simulink model "cascadedadrnmpcnofuzzyobs"  (R2024b)
settings: Solver=FixedStepDiscrete  StartTime=0.0  StopTime=80000  FixedStep=0.05  RelTol=1e-3  EnableMultiTasking=on
StartFcn:
  | tic
StopFcn:
  | ttt2=toc
undefined symbols (not defined in the file or in its folder): Force, Torque
libraries: robotlib x12
settings Model: SimulationMode=accelerator  PacingRate=0.010000  Creator=xiejingdong  LastModifiedBy=lenovo
settings SolverCC: ConcurrentTasks=on  AlgebraicLoopSolver=TrustRegion
settings DataIOCC: ReturnWorkspaceOutputs=off
settings DebuggingCC: UnconnectedInputMsg=warning  UnconnectedOutputMsg=warning  UnconnectedLineMsg=warning
settings ModelReferenceCC: EnableRefExpFcnMdlSchedulingChecks=on
settings RTWCC: GPUComputeCapability=3.5  DLArmComputeVersion=19.05

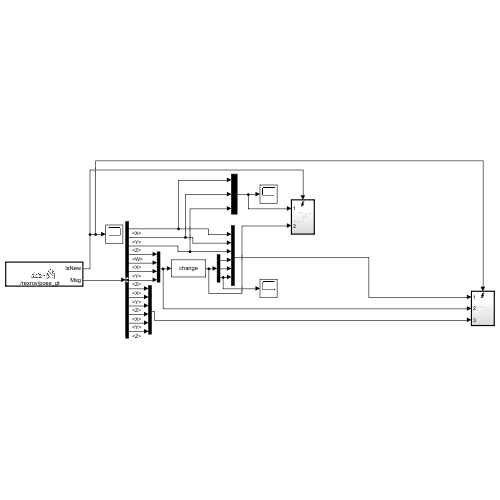
[thumbnail: Simulink's stored preview of the top-level diagram]
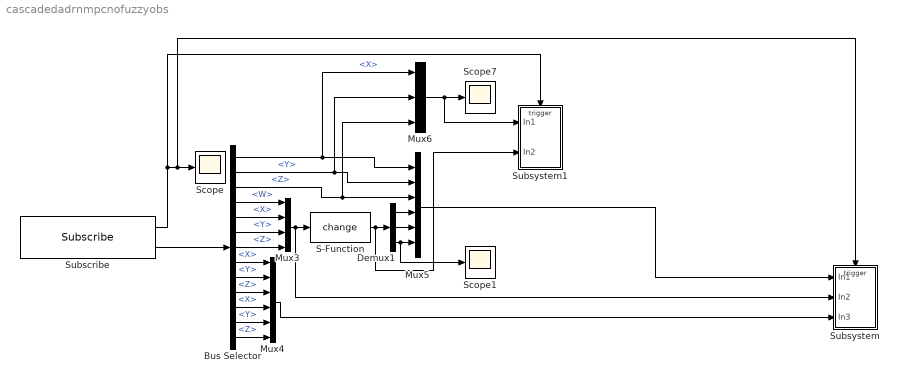
== system cascadedadrnmpcnofuzzyobs ==
  Bus Selector : BusSelector  OutputSignals=Pose.Pose.Position.X,Pose.Pose.Position.Y,Pose.Pose.Position.Z,Pose.Pose.Orientation.W,Pose.Pose.Orientation.X,Pose.Pose.Orientation.Y,Pose.Pose.Orientation.Z,Twist.Twist.Linear.X,Twist.Twist.Linear.Y,Twist.Twist.Linear.Z,Twist.Twist.Angular.X,Twist.Twist.Angular.Y,Twist.Twist.Angular.Z
  Demux1 : Demux  Outputs=3
  Mux3 : Mux
  Mux4 : Mux  Inputs=6
  Mux5 : Mux  Inputs=6
  Mux6 : Mux  Inputs=3
  S-Function : S-Function  FunctionName=change  SFunctionDeploymentMode=off  EnableBusSupport=off
  Scope : Scope
  Scope1 : Scope
  Scope7 : Scope
  Subscribe : robotlib/Subscribe  topicSource=Select from ROS network  topic=/rexrov/pose_gt  messageType=nav_msgs/Odometry  SampleTime=-1  legacyBusStruct=off  messageQueueLength=1
  Subsystem : Subsystem
  Subsystem1 : Subsystem
  wires:
  Subscribe/1 -> Subsystem1/Trigger, Subsystem/Trigger, Scope/1
  Subscribe/2 -> Bus Selector/1
  Bus Selector/4 -> Mux3/1  "<W>"
  Bus Selector/5 -> Mux3/2  "<X>"
  Bus Selector/6 -> Mux3/3  "<Y>"
  Bus Selector/7 -> Mux3/4  "<Z>"
  Bus Selector/8 -> Mux4/1  "<X>"
  Bus Selector/11 -> Mux4/4  "<X>"
  Bus Selector/10 -> Mux4/3  "<Z>"
  Bus Selector/9 -> Mux4/2  "<Y>"
  Bus Selector/12 -> Mux4/5  "<Y>"
  Bus Selector/13 -> Mux4/6  "<Z>"
  Mux3/1 -> Subsystem/2(In2), S-Function/1
  S-Function/1 -> Subsystem1/2(In2), Demux1/1
  Demux1/3 -> Scope1/1, Mux5/6
  Demux1/2 -> Mux5/5
  Demux1/1 -> Mux5/4
  Bus Selector/3 -> Mux6/3, Mux5/3  "<Z>"
  Bus Selector/2 -> Mux6/2, Mux5/2  "<Y>"
  Bus Selector/1 -> Mux6/1, Mux5/1  "<X>"
  Mux6/1 -> Subsystem1/1(In1), Scope7/1
  Mux5/1 -> Subsystem/1(In1)
  Mux4/1 -> Subsystem/3(In3)

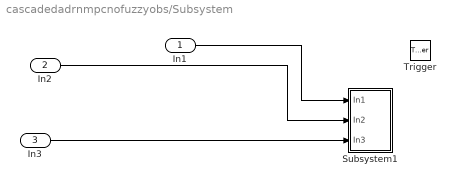
== system cascadedadrnmpcnofuzzyobs/Subsystem ==
  In1 : Inport
  In2 : Inport  Port=2
  In3 : Inport  Port=3
  Trigger : TriggerPort  VariantControl=(inherit)  PortDimensions=1
  Subsystem1 : Subsystem
  wires:
  In1/1 -> Subsystem1/1(In1)
  In2/1 -> Subsystem1/2(In2)
  In3/1 -> Subsystem1/3(In3)

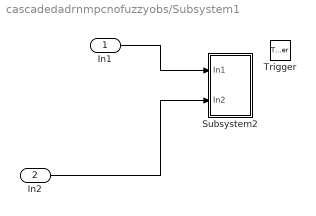
== system cascadedadrnmpcnofuzzyobs/Subsystem1 ==
  In1 : Inport
  In2 : Inport  Port=2
  Trigger : TriggerPort  VariantControl=(inherit)  PortDimensions=1
  Subsystem2 : Subsystem
  wires:
  In2/1 -> Subsystem2/2(In2)
  In1/1 -> Subsystem2/1(In1)

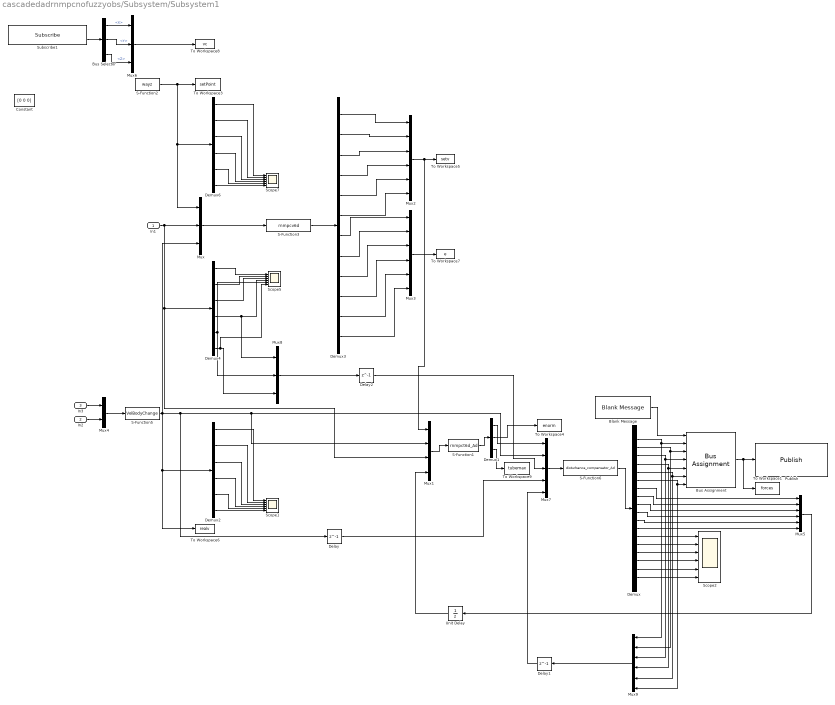
== system cascadedadrnmpcnofuzzyobs/Subsystem/Subsystem1 ==
  In1 : Inport
  In2 : Inport  Port=2
  In3 : Inport  Port=3
  Blank Message : robotlib/Blank Message  messageClass=Message  entityType=geometry_msgs/Wrench  messageType=geometry_msgs/Wrench  SampleTime=-1  legacyBusStruct=off
  Bus Assignment : BusAssignment  AssignedSignals=Force.X,Force.Y,Force.Z,Torque.X,Torque.Y,Torque.Z
  Bus Selector : BusSelector  OutputSignals=Twist.Linear.X,Twist.Linear.Y,Twist.Linear.Z
  Constant : Constant  Value=[0 0 0]
  Delay : Delay  DelayLength=1  InitialCondition=0
  Delay1 : Delay  DelayLength=1  InitialCondition=0
  Delay2 : Delay  DelayLength=1  InitialCondition=0
  Demux : Demux  Outputs=18
  Demux1 : Demux  Outputs=3
  Demux2 : Demux  Outputs=6
  Demux3 : Demux  Outputs=12
  Demux4 : Demux  Outputs=6
  Demux6 : Demux  Outputs=6
  Mux : Mux  Inputs=3
  Mux1 : Mux
  Mux{2..3,5,9} (4 alike) : Mux  Inputs=6
  Mux4 : Mux  Inputs=2
  Mux6 : Mux  Inputs=3
  Mux7 : Mux  Inputs=5
  Mux8 : Mux  Inputs=3
  Publish : robotlib/Publish  topicSource=Select from ROS network  topic=/rexrov/thruster_manager/input  messageType=geometry_msgs/Wrench  legacyBusStruct=off  messageQueueLength=1
  S-Function1 : S-Function  FunctionName=rnmpct6d_Ad  Parameters=0  SFunctionDeploymentMode=off  EnableBusSupport=off
  S-Function2 : S-Function  FunctionName=wayz  SFunctionDeploymentMode=off  EnableBusSupport=off
  S-Function3 : S-Function  FunctionName=rnmpcv6d  Parameters=0  SFunctionDeploymentMode=off  EnableBusSupport=off
  S-Function5 : S-Function  FunctionName=VelBodyChange  SFunctionDeploymentMode=off  EnableBusSupport=off
  S-Function6 : S-Function  FunctionName=disturbance_compensator_Ad  SFunctionDeploymentMode=off  EnableBusSupport=off
  Scope{1..2,5,7} (4 alike) : Scope  NumInputPorts=6
  Subscribe1 : robotlib/Subscribe  topicSource=Select from ROS network  topic=/hydrodynamics/current_velocity  messageType=geometry_msgs/TwistStamped  SampleTime=-1  legacyBusStruct=off  messageQueueLength=1
  To Workspace1 : ToWorkspace  VariableName=forces  SaveFormat=Timeseries  SampleTime=-1
  To Workspace3 : ToWorkspace  VariableName=setPoint  SampleTime=-1
      settings: Save2DSignal=2-D array (concatenate along first dimension)
  To Workspace4 : ToWorkspace  VariableName=enorm  SampleTime=-1
      settings: Save2DSignal=2-D array (concatenate along first dimension)
  To Workspace5 : ToWorkspace  VariableName=setv  SampleTime=-1
      settings: Save2DSignal=2-D array (concatenate along first dimension)
  To Workspace6 : ToWorkspace  VariableName=realv  SampleTime=-1
      settings: Save2DSignal=2-D array (concatenate along first dimension)
  To Workspace7 : ToWorkspace  VariableName=e  SampleTime=-1
      settings: Save2DSignal=2-D array (concatenate along first dimension)
  To Workspace8 : ToWorkspace  VariableName=vc  SampleTime=-1
      settings: Save2DSignal=2-D array (concatenate along first dimension)
  To Workspace9 : ToWorkspace  VariableName=tubemax  SampleTime=-1
      settings: Save2DSignal=2-D array (concatenate along first dimension)
  Unit Delay : UnitDelay  SampleTime=-1  HasFrameUpgradeWarning=on
  wires:
  Mux/1 -> S-Function3/1
  Demux6/4 -> Scope7/4
  Subscribe1/2 -> Bus Selector/1
  Demux3/4 -> Mux2/4
  In3/1 -> Mux4/1
  Bus Selector/3 -> Mux6/3  "<Z>"
  Demux3/10 -> Mux3/4
  Demux3/2 -> Mux2/2
  Demux2/2 -> Scope1/2
  In2/1 -> Mux4/2
  Bus Selector/1 -> Mux6/1  "<X>"
  Demux3/3 -> Mux2/3
  Demux2/3 -> Scope1/3
  Bus Selector/2 -> Mux6/2  "<Y>"
  Mux4/1 -> S-Function5/1
  Mux6/1 -> To Workspace8/1
  S-Function5/1 -> To Workspace6/1, Demux2/1, Mux7/2, Mux1/2, Delay/1, Mux/3
  S-Function2/1 -> Mux/1, Demux6/1, To Workspace3/1
  Demux3/8 -> Mux3/2
  In1/1 -> Demux4/1, Mux1/3, Mux/2
  Demux6/1 -> Scope7/1
  Demux6/2 -> Scope7/2
  Demux2/5 -> Scope1/5
  Demux4/3 -> Scope5/3
  Demux6/3 -> Scope7/3
  Demux6/5 -> Scope7/5
  Demux6/6 -> Scope7/6
  Demux4/1 -> Scope5/1
  Mux1/1 -> S-Function1/1
  Demux4/2 -> Scope5/2
  Demux4/4 -> Scope5/4, Mux8/1
  Demux4/5 -> Scope5/5, Mux8/2
  Demux4/6 -> Scope5/6, Mux8/3
  Demux3/9 -> Mux3/3
  Demux3/1 -> Mux2/1
  Demux2/1 -> Scope1/1
  Demux3/12 -> Mux3/6
  Demux2/4 -> Scope1/4
  Demux3/6 -> Mux2/6
  Demux2/6 -> Scope1/6
  S-Function3/1 -> Demux3/1
  Mux8/1 -> Delay2/1
  Demux3/5 -> Mux2/5
  Demux3/7 -> Mux3/1
  Demux3/11 -> Mux3/5
  S-Function1/1 -> Demux1/1
  Delay/1 -> Mux7/4
  Mux3/1 -> To Workspace7/1
  Mux2/1 -> Mux1/1, To Workspace5/1
  Mux7/1 -> S-Function6/1
  Blank Message/1 -> Bus Assignment/1
  Bus Assignment/1 -> Publish/1, To Workspace1/1
  Demux1/1 -> Mux7/1
  Demux1/2 -> To Workspace4/1
  S-Function6/1 -> Demux/1
  Demux/2 -> Mux9/2, Bus Assignment/3
  Delay1/1 -> Mux7/5
  Demux/6 -> Mux9/6, Bus Assignment/7
  Demux/5 -> Mux9/5, Bus Assignment/6
  Demux/1 -> Mux9/1, Bus Assignment/2
  Demux/3 -> Mux9/3, Bus Assignment/4
  Demux/4 -> Mux9/4, Bus Assignment/5
  Mux9/1 -> Delay1/1
  Demux/9 -> Mux5/3
  Demux/10 -> Mux5/4
  Demux/11 -> Mux5/5
  Demux/12 -> Mux5/6
  Demux/7 -> Mux5/1
  Demux/8 -> Mux5/2
  Mux5/1 -> Unit Delay/1
  Unit Delay/1 -> Mux1/4
  Demux1/3 -> To Workspace9/1
  Delay2/1 -> Mux7/3
  Demux/13 -> Scope2/1
  Demux/14 -> Scope2/2
  Demux/15 -> Scope2/3
  Demux/16 -> Scope2/4
  Demux/17 -> Scope2/5
  Demux/18 -> Scope2/6

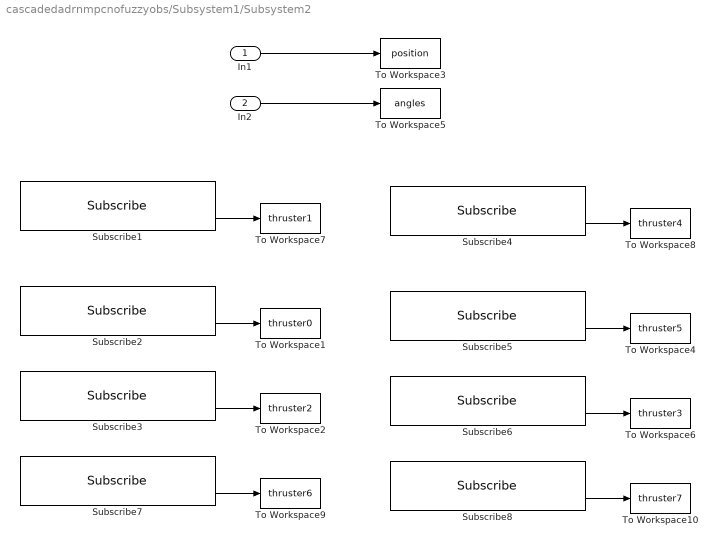
== system cascadedadrnmpcnofuzzyobs/Subsystem1/Subsystem2 ==
  In1 : Inport
  In2 : Inport  Port=2
  Subscribe1 : robotlib/Subscribe  topicSource=Select from ROS network  topic=/rexrov/thrusters/1/thrust_wrench  messageType=geometry_msgs/WrenchStamped  SampleTime=-1  legacyBusStruct=off  messageQueueLength=1
  Subscribe2 : robotlib/Subscribe  topicSource=Select from ROS network  topic=/rexrov/thrusters/0/thrust_wrench  messageType=geometry_msgs/WrenchStamped  SampleTime=-1  legacyBusStruct=off  messageQueueLength=1
  Subscribe3 : robotlib/Subscribe  topicSource=Select from ROS network  topic=/rexrov/thrusters/2/thrust_wrench  messageType=geometry_msgs/WrenchStamped  SampleTime=-1  legacyBusStruct=off  messageQueueLength=1
  Subscribe4 : robotlib/Subscribe  topicSource=Select from ROS network  topic=/rexrov/thrusters/4/thrust_wrench  messageType=geometry_msgs/WrenchStamped  SampleTime=-1  legacyBusStruct=off  messageQueueLength=1
  Subscribe5 : robotlib/Subscribe  topicSource=Select from ROS network  topic=/rexrov/thrusters/5/thrust_wrench  messageType=geometry_msgs/WrenchStamped  SampleTime=-1  legacyBusStruct=off  messageQueueLength=1
  Subscribe6 : robotlib/Subscribe  topicSource=Select from ROS network  topic=/rexrov/thrusters/3/thrust_wrench  messageType=geometry_msgs/WrenchStamped  SampleTime=-1  legacyBusStruct=off  messageQueueLength=1
  Subscribe7 : robotlib/Subscribe  topicSource=Select from ROS network  topic=/rexrov/thrusters/6/thrust_wrench  messageType=geometry_msgs/WrenchStamped  SampleTime=-1  legacyBusStruct=off  messageQueueLength=1
  Subscribe8 : robotlib/Subscribe  topicSource=Select from ROS network  topic=/rexrov/thrusters/7/thrust_wrench  messageType=geometry_msgs/WrenchStamped  SampleTime=-1  legacyBusStruct=off  messageQueueLength=1
  To Workspace1 : ToWorkspace  VariableName=thruster0  SaveFormat=Timeseries  SampleTime=-1
  To Workspace10 : ToWorkspace  VariableName=thruster7  SaveFormat=Timeseries  SampleTime=-1
  To Workspace2 : ToWorkspace  VariableName=thruster2  SaveFormat=Timeseries  SampleTime=-1
  To Workspace3 : ToWorkspace  VariableName=position  SaveFormat=Timeseries  SampleTime=-1
  To Workspace4 : ToWorkspace  VariableName=thruster5  SaveFormat=Timeseries  SampleTime=-1
  To Workspace5 : ToWorkspace  VariableName=angles  SaveFormat=Timeseries  SampleTime=-1
  To Workspace6 : ToWorkspace  VariableName=thruster3  SaveFormat=Timeseries  SampleTime=-1
  To Workspace7 : ToWorkspace  VariableName=thruster1  SaveFormat=Timeseries  SampleTime=-1
  To Workspace8 : ToWorkspace  VariableName=thruster4  SaveFormat=Timeseries  SampleTime=-1
  To Workspace9 : ToWorkspace  VariableName=thruster6  SaveFormat=Timeseries  SampleTime=-1
  wires:
  Subscribe5/2 -> To Workspace4/1
  Subscribe6/2 -> To Workspace6/1
  Subscribe8/2 -> To Workspace10/1
  Subscribe3/2 -> To Workspace2/1
  In2/1 -> To Workspace5/1
  In1/1 -> To Workspace3/1
  Subscribe4/2 -> To Workspace8/1
  Subscribe1/2 -> To Workspace7/1
  Subscribe7/2 -> To Workspace9/1
  Subscribe2/2 -> To Workspace1/1
